simulink model "Parachute"  (R2025b)
settings: Solver=VariableStepAuto  StartTime=0.0  StopTime=40.0  RelTol=1e-3
libraries: simulink x1
settings Model: Creator=ssokolov  LastModifiedBy=ssokolov

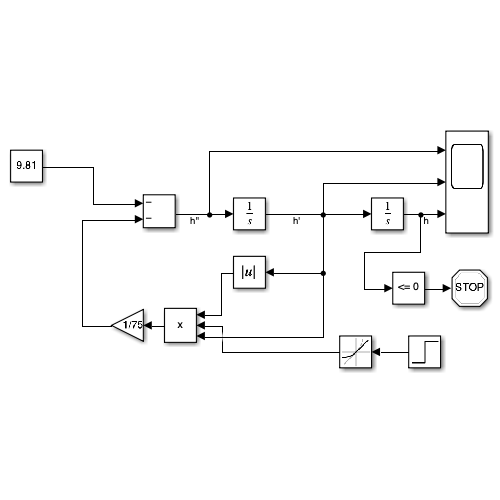
[thumbnail: Simulink's stored preview of the top-level diagram]
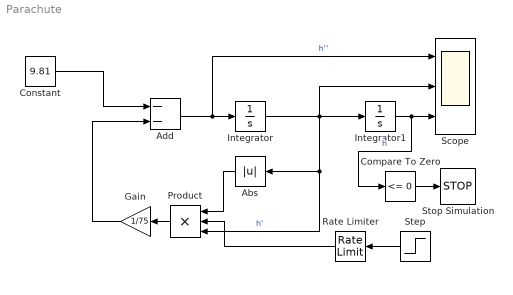
== system Parachute ==
  Abs : Abs  SaturateOnIntegerOverflow=off
  Add : Sum  Inputs=--
  Compare To Zero : simulink/Logic and Bit Operations/Compare To Zero  relop=<=  OutDataTypeStr=boolean
  Constant : Constant  Value=9.81
  Gain : Gain  Gain=1/75
  Integrator : Integrator
  Integrator1 : Integrator  InitialCondition=600
  Product : Product  Inputs=3
  Rate Limiter : RateLimiter  RisingSlewLimit=8  SampleTimeMode=inherited
  Scope : Scope  NumInputPorts=3
      settings: ActiveDisplayYMinimum=-69.002007745668  ActiveDisplayYMaximum=154.15680565143717
  Step : Step  Time=20  Before=1  After=25  SampleTime=0
  Stop Simulation : Stop
  wires:
  Integrator/1 -> Scope/2, Integrator1/1, Product/3, Abs/1  "h'"
  Add/1 -> Scope/1, Integrator/1  "h''"
  Integrator1/1 -> Compare To Zero/1, Scope/3  "h"
  Constant/1 -> Add/1
  Abs/1 -> Product/1
  Step/1 -> Rate Limiter/1
  Product/1 -> Gain/1
  Rate Limiter/1 -> Product/2
  Gain/1 -> Add/2
  Compare To Zero/1 -> Stop Simulation/1
